simulink library "xrbsComm_r4"  (Simulink 7.1)
PreLoadFcn:
  | warning('off','MATLAB:mex:deprecatedExtension');xlmeta;com.xilinx.sysgen.util.StrategyUtil.loadAllStrategyNames();
undefined symbols (not defined in the file or in its folder): calc_path_data, gcbh, mfcm_matrix_rom, oct2dec, xlBlockLoadCallback
libraries: xbsIndex_r4 x851, mfcm_block_lib_v1 x5, xrbsComm_r4 x1, mfcm_misc_lib_v1 x1
(part 6 of 8)

== system xrbsComm_r4/White Gaussian  Noise Generator/Box-Muller1/f/lfsr_17_2/x1/ASR ==
  din : Inport  OutDataType=sfix(16)  OutScaling=2^0
  Addressable Shift Register : xbsIndex_r4/Addressable Shift Register  infer_latency=off  depth=asr_length  initVector=init  en=off  dbl_ovrd=off  use_behavioral_HDL=off  use_rpm=off  block_type=addrsr
      settings: infoedit="Delay of configurable length.  Any element in the delay line can be addressed and driven onto the output port.<P><P>Hardware notes: Implemented using SRL16s.  If a Virtex-II device is used, multiple SRLC16s are cascaded together."  xl_area=[0, 0, 0, 0, 0, 0, 0]  block_version=VER_STRING_GOES_HERE
  Constant1 : xbsIndex_r4/Constant  arith_type=Unsigned  const=asr_length-1  n_bits=size(dec2bin(asr_length-1),2)  bin_pt=0  explicit_period=off  period=1  equ=P=C  opselect=C  inp2=PCIN>>17  opr=+  inp1=P  carry=CIN  dbl_ovrd=off  block_type=constant
      settings: block_version=VER_STRING_GOES_HERE
  dout : Outport  OutDataType=sfix(16)  OutScaling=2^0
  wires:
  Constant1/1 -> Addressable Shift Register/2
  Addressable Shift Register/1 -> dout/1
  din/1 -> Addressable Shift Register/1

== system xrbsComm_r4/White Gaussian  Noise Generator/Box-Muller1/f/lfsr_17_2/x5/ASR ==
  din : Inport  OutDataType=sfix(16)  OutScaling=2^0
  Addressable Shift Register : xbsIndex_r4/Addressable Shift Register  infer_latency=off  depth=asr_length  initVector=init  en=off  dbl_ovrd=off  use_behavioral_HDL=off  use_rpm=off  block_type=addrsr
      settings: infoedit="Delay of configurable length.  Any element in the delay line can be addressed and driven onto the output port.<P><P>Hardware notes: Implemented using SRL16s.  If a Virtex-II device is used, multiple SRLC16s are cascaded together."  xl_area=[0, 0, 0, 0, 0, 0, 0]  block_version=VER_STRING_GOES_HERE
  Constant : xbsIndex_r4/Constant  arith_type=Unsigned  const=asr_length-1  n_bits=size(dec2bin(asr_length-1),2)  bin_pt=0  explicit_period=off  period=1  equ=P=C  opselect=C  inp2=PCIN>>17  opr=+  inp1=P  carry=CIN  dbl_ovrd=off  block_type=constant
      settings: block_version=VER_STRING_GOES_HERE
  dout : Outport  OutDataType=sfix(16)  OutScaling=2^0
  wires:
  Constant/1 -> Addressable Shift Register/2
  Addressable Shift Register/1 -> dout/1
  din/1 -> Addressable Shift Register/1

== system xrbsComm_r4/White Gaussian  Noise Generator/Box-Muller1/f/lfsr_17_2/x6/ASR ==
  din : Inport  OutDataType=sfix(16)  OutScaling=2^0
  Addressable Shift Register : xbsIndex_r4/Addressable Shift Register  infer_latency=off  depth=asr_length  initVector=init  en=off  dbl_ovrd=off  use_behavioral_HDL=off  use_rpm=off  block_type=addrsr
      settings: infoedit="Delay of configurable length.  Any element in the delay line can be addressed and driven onto the output port.<P><P>Hardware notes: Implemented using SRL16s.  If a Virtex-II device is used, multiple SRLC16s are cascaded together."  xl_area=[0, 0, 0, 0, 0, 0, 0]  block_version=VER_STRING_GOES_HERE
  Constant : xbsIndex_r4/Constant  arith_type=Unsigned  const=asr_length-1  n_bits=size(dec2bin(asr_length-1),2)  bin_pt=0  explicit_period=off  period=1  equ=P=C  opselect=C  inp2=PCIN>>17  opr=+  inp1=P  carry=CIN  dbl_ovrd=off  block_type=constant
      settings: block_version=VER_STRING_GOES_HERE
  dout : Outport  OutDataType=sfix(16)  OutScaling=2^0
  wires:
  Constant/1 -> Addressable Shift Register/2
  Addressable Shift Register/1 -> dout/1
  din/1 -> Addressable Shift Register/1

== system xrbsComm_r4/White Gaussian  Noise Generator/Box-Muller1/f/lfsr_17_2/x7/ASR ==
  din : Inport  OutDataType=sfix(16)  OutScaling=2^0
  Addressable Shift Register : xbsIndex_r4/Addressable Shift Register  infer_latency=off  depth=asr_length  initVector=init  en=off  dbl_ovrd=off  use_behavioral_HDL=off  use_rpm=off  block_type=addrsr
      settings: infoedit="Delay of configurable length.  Any element in the delay line can be addressed and driven onto the output port.<P><P>Hardware notes: Implemented using SRL16s.  If a Virtex-II device is used, multiple SRLC16s are cascaded together."  xl_area=[0, 0, 0, 0, 0, 0, 0]  block_version=VER_STRING_GOES_HERE
  Constant : xbsIndex_r4/Constant  arith_type=Unsigned  const=asr_length-1  n_bits=size(dec2bin(asr_length-1),2)  bin_pt=0  explicit_period=off  period=1  equ=P=C  opselect=C  inp2=PCIN>>17  opr=+  inp1=P  carry=CIN  dbl_ovrd=off  block_type=constant
      settings: block_version=VER_STRING_GOES_HERE
  dout : Outport  OutDataType=sfix(16)  OutScaling=2^0
  wires:
  Constant/1 -> Addressable Shift Register/2
  Addressable Shift Register/1 -> dout/1
  din/1 -> Addressable Shift Register/1

== system xrbsComm_r4/White Gaussian  Noise Generator/Box-Muller1/f/lfsr_25_1/x1/ASR ==
  din : Inport  OutDataType=sfix(16)  OutScaling=2^0
  Addressable Shift Register : xbsIndex_r4/Addressable Shift Register  infer_latency=off  depth=asr_length  initVector=init  en=off  dbl_ovrd=off  use_behavioral_HDL=off  use_rpm=off  block_type=addrsr
      settings: infoedit="Delay of configurable length.  Any element in the delay line can be addressed and driven onto the output port.<P><P>Hardware notes: Implemented using SRL16s.  If a Virtex-II device is used, multiple SRLC16s are cascaded together."  xl_area=[0, 0, 0, 0, 0, 0, 0]  block_version=VER_STRING_GOES_HERE
  Constant1 : xbsIndex_r4/Constant  arith_type=Unsigned  const=asr_length-1  n_bits=size(dec2bin(asr_length-1),2)  bin_pt=0  explicit_period=off  period=1  equ=P=C  opselect=C  inp2=PCIN>>17  opr=+  inp1=P  carry=CIN  dbl_ovrd=off  block_type=constant
      settings: block_version=VER_STRING_GOES_HERE
  dout : Outport  OutDataType=sfix(16)  OutScaling=2^0
  wires:
  Constant1/1 -> Addressable Shift Register/2
  Addressable Shift Register/1 -> dout/1
  din/1 -> Addressable Shift Register/1

== system xrbsComm_r4/White Gaussian  Noise Generator/Box-Muller1/f/lfsr_25_1/x5/ASR ==
  din : Inport  OutDataType=sfix(16)  OutScaling=2^0
  Addressable Shift Register : xbsIndex_r4/Addressable Shift Register  infer_latency=off  depth=asr_length  initVector=init  en=off  dbl_ovrd=off  use_behavioral_HDL=off  use_rpm=off  block_type=addrsr
      settings: infoedit="Delay of configurable length.  Any element in the delay line can be addressed and driven onto the output port.<P><P>Hardware notes: Implemented using SRL16s.  If a Virtex-II device is used, multiple SRLC16s are cascaded together."  xl_area=[0, 0, 0, 0, 0, 0, 0]  block_version=VER_STRING_GOES_HERE
  Constant1 : xbsIndex_r4/Constant  arith_type=Unsigned  const=asr_length-1  n_bits=size(dec2bin(asr_length-1),2)  bin_pt=0  explicit_period=off  period=1  equ=P=C  opselect=C  inp2=PCIN>>17  opr=+  inp1=P  carry=CIN  dbl_ovrd=off  block_type=constant
      settings: block_version=VER_STRING_GOES_HERE
  dout : Outport  OutDataType=sfix(16)  OutScaling=2^0
  wires:
  Constant1/1 -> Addressable Shift Register/2
  Addressable Shift Register/1 -> dout/1
  din/1 -> Addressable Shift Register/1

== system xrbsComm_r4/White Gaussian  Noise Generator/Box-Muller1/f/lfsr_25_1/x6/ASR ==
  din : Inport  OutDataType=sfix(16)  OutScaling=2^0
  Addressable Shift Register : xbsIndex_r4/Addressable Shift Register  infer_latency=off  depth=asr_length  initVector=init  en=off  dbl_ovrd=off  use_behavioral_HDL=off  use_rpm=off  block_type=addrsr
      settings: infoedit="Delay of configurable length.  Any element in the delay line can be addressed and driven onto the output port.<P><P>Hardware notes: Implemented using SRL16s.  If a Virtex-II device is used, multiple SRLC16s are cascaded together."  xl_area=[0, 0, 0, 0, 0, 0, 0]  block_version=VER_STRING_GOES_HERE
  Constant1 : xbsIndex_r4/Constant  arith_type=Unsigned  const=asr_length-1  n_bits=size(dec2bin(asr_length-1),2)  bin_pt=0  explicit_period=off  period=1  equ=P=C  opselect=C  inp2=PCIN>>17  opr=+  inp1=P  carry=CIN  dbl_ovrd=off  block_type=constant
      settings: block_version=VER_STRING_GOES_HERE
  dout : Outport  OutDataType=sfix(16)  OutScaling=2^0
  wires:
  Constant1/1 -> Addressable Shift Register/2
  Addressable Shift Register/1 -> dout/1
  din/1 -> Addressable Shift Register/1

== system xrbsComm_r4/White Gaussian  Noise Generator/Box-Muller1/f/lfsr_25_1/x7/ASR ==
  din : Inport  OutDataType=sfix(16)  OutScaling=2^0
  Addressable Shift Register : xbsIndex_r4/Addressable Shift Register  infer_latency=off  depth=asr_length  initVector=init  en=off  dbl_ovrd=off  use_behavioral_HDL=off  use_rpm=off  block_type=addrsr
      settings: infoedit="Delay of configurable length.  Any element in the delay line can be addressed and driven onto the output port.<P><P>Hardware notes: Implemented using SRL16s.  If a Virtex-II device is used, multiple SRLC16s are cascaded together."  xl_area=[0, 0, 0, 0, 0, 0, 0]  block_version=VER_STRING_GOES_HERE
  Constant1 : xbsIndex_r4/Constant  arith_type=Unsigned  const=asr_length-1  n_bits=size(dec2bin(asr_length-1),2)  bin_pt=0  explicit_period=off  period=1  equ=P=C  opselect=C  inp2=PCIN>>17  opr=+  inp1=P  carry=CIN  dbl_ovrd=off  block_type=constant
      settings: block_version=VER_STRING_GOES_HERE
  dout : Outport  OutDataType=sfix(16)  OutScaling=2^0
  wires:
  Constant1/1 -> Addressable Shift Register/2
  Addressable Shift Register/1 -> dout/1
  din/1 -> Addressable Shift Register/1

== system xrbsComm_r4/White Gaussian  Noise Generator/Box-Muller1/f/lfsr_29_2/x5/ASR ==
  din : Inport  OutDataType=sfix(16)  OutScaling=2^0
  Addressable Shift Register : xbsIndex_r4/Addressable Shift Register  infer_latency=off  depth=asr_length  initVector=init  en=off  dbl_ovrd=off  use_behavioral_HDL=off  use_rpm=off  block_type=addrsr
      settings: infoedit="Delay of configurable length.  Any element in the delay line can be addressed and driven onto the output port.<P><P>Hardware notes: Implemented using SRL16s.  If a Virtex-II device is used, multiple SRLC16s are cascaded together."  xl_area=[0, 0, 0, 0, 0, 0, 0]  block_version=VER_STRING_GOES_HERE
  Constant1 : xbsIndex_r4/Constant  arith_type=Unsigned  const=asr_length-1  n_bits=size(dec2bin(asr_length-1),2)  bin_pt=0  explicit_period=off  period=1  equ=P=C  opselect=C  inp2=PCIN>>17  opr=+  inp1=P  carry=CIN  dbl_ovrd=off  block_type=constant
      settings: block_version=VER_STRING_GOES_HERE
  dout : Outport  OutDataType=sfix(16)  OutScaling=2^0
  wires:
  Constant1/1 -> Addressable Shift Register/2
  Addressable Shift Register/1 -> dout/1
  din/1 -> Addressable Shift Register/1

== system xrbsComm_r4/White Gaussian  Noise Generator/Box-Muller1/f/lfsr_29_2/x6/ASR ==
  din : Inport  OutDataType=sfix(16)  OutScaling=2^0
  Addressable Shift Register : xbsIndex_r4/Addressable Shift Register  infer_latency=off  depth=asr_length  initVector=init  en=off  dbl_ovrd=off  use_behavioral_HDL=off  use_rpm=off  block_type=addrsr
      settings: infoedit="Delay of configurable length.  Any element in the delay line can be addressed and driven onto the output port.<P><P>Hardware notes: Implemented using SRL16s.  If a Virtex-II device is used, multiple SRLC16s are cascaded together."  xl_area=[0, 0, 0, 0, 0, 0, 0]  block_version=VER_STRING_GOES_HERE
  Constant1 : xbsIndex_r4/Constant  arith_type=Unsigned  const=asr_length-1  n_bits=size(dec2bin(asr_length-1),2)  bin_pt=0  explicit_period=off  period=1  equ=P=C  opselect=C  inp2=PCIN>>17  opr=+  inp1=P  carry=CIN  dbl_ovrd=off  block_type=constant
      settings: block_version=VER_STRING_GOES_HERE
  dout : Outport  OutDataType=sfix(16)  OutScaling=2^0
  wires:
  Constant1/1 -> Addressable Shift Register/2
  Addressable Shift Register/1 -> dout/1
  din/1 -> Addressable Shift Register/1

== system xrbsComm_r4/White Gaussian  Noise Generator/Box-Muller1/f/lfsr_29_2/x7/ASR ==
  din : Inport  OutDataType=sfix(16)  OutScaling=2^0
  Addressable Shift Register : xbsIndex_r4/Addressable Shift Register  infer_latency=off  depth=asr_length  initVector=init  en=off  dbl_ovrd=off  use_behavioral_HDL=off  use_rpm=off  block_type=addrsr
      settings: infoedit="Delay of configurable length.  Any element in the delay line can be addressed and driven onto the output port.<P><P>Hardware notes: Implemented using SRL16s.  If a Virtex-II device is used, multiple SRLC16s are cascaded together."  xl_area=[0, 0, 0, 0, 0, 0, 0]  block_version=VER_STRING_GOES_HERE
  Constant1 : xbsIndex_r4/Constant  arith_type=Unsigned  const=asr_length-1  n_bits=size(dec2bin(asr_length-1),2)  bin_pt=0  explicit_period=off  period=1  equ=P=C  opselect=C  inp2=PCIN>>17  opr=+  inp1=P  carry=CIN  dbl_ovrd=off  block_type=constant
      settings: block_version=VER_STRING_GOES_HERE
  dout : Outport  OutDataType=sfix(16)  OutScaling=2^0
  wires:
  Constant1/1 -> Addressable Shift Register/2
  Addressable Shift Register/1 -> dout/1
  din/1 -> Addressable Shift Register/1

== system xrbsComm_r4/White Gaussian  Noise Generator/Box-Muller1/f/lfsr_29_2/x8/ASR ==
  din : Inport  OutDataType=sfix(16)  OutScaling=2^0
  Addressable Shift Register : xbsIndex_r4/Addressable Shift Register  infer_latency=off  depth=asr_length  initVector=init  en=off  dbl_ovrd=off  use_behavioral_HDL=off  use_rpm=off  block_type=addrsr
      settings: infoedit="Delay of configurable length.  Any element in the delay line can be addressed and driven onto the output port.<P><P>Hardware notes: Implemented using SRL16s.  If a Virtex-II device is used, multiple SRLC16s are cascaded together."  xl_area=[0, 0, 0, 0, 0, 0, 0]  block_version=VER_STRING_GOES_HERE
  Constant1 : xbsIndex_r4/Constant  arith_type=Unsigned  const=asr_length-1  n_bits=size(dec2bin(asr_length-1),2)  bin_pt=0  explicit_period=off  period=1  equ=P=C  opselect=C  inp2=PCIN>>17  opr=+  inp1=P  carry=CIN  dbl_ovrd=off  block_type=constant
      settings: block_version=VER_STRING_GOES_HERE
  dout : Outport  OutDataType=sfix(16)  OutScaling=2^0
  wires:
  Constant1/1 -> Addressable Shift Register/2
  Addressable Shift Register/1 -> dout/1
  din/1 -> Addressable Shift Register/1

== system xrbsComm_r4/White Gaussian  Noise Generator/Box-Muller1/f/lfsr_31_2/x5/ASR ==
  din : Inport  OutDataType=sfix(16)  OutScaling=2^0
  Addressable Shift Register : xbsIndex_r4/Addressable Shift Register  infer_latency=off  depth=asr_length  initVector=init  en=off  dbl_ovrd=off  use_behavioral_HDL=off  use_rpm=off  block_type=addrsr
      settings: infoedit="Delay of configurable length.  Any element in the delay line can be addressed and driven onto the output port.<P><P>Hardware notes: Implemented using SRL16s.  If a Virtex-II device is used, multiple SRLC16s are cascaded together."  xl_area=[0, 0, 0, 0, 0, 0, 0]  block_version=VER_STRING_GOES_HERE
  Constant1 : xbsIndex_r4/Constant  arith_type=Unsigned  const=asr_length-1  n_bits=size(dec2bin(asr_length-1),2)  bin_pt=0  explicit_period=off  period=1  equ=P=C  opselect=C  inp2=PCIN>>17  opr=+  inp1=P  carry=CIN  dbl_ovrd=off  block_type=constant
      settings: block_version=VER_STRING_GOES_HERE
  dout : Outport  OutDataType=sfix(16)  OutScaling=2^0
  wires:
  Constant1/1 -> Addressable Shift Register/2
  Addressable Shift Register/1 -> dout/1
  din/1 -> Addressable Shift Register/1

== system xrbsComm_r4/White Gaussian  Noise Generator/Box-Muller1/f/lfsr_31_2/x6/ASR ==
  din : Inport  OutDataType=sfix(16)  OutScaling=2^0
  Addressable Shift Register : xbsIndex_r4/Addressable Shift Register  infer_latency=off  depth=asr_length  initVector=init  en=off  dbl_ovrd=off  use_behavioral_HDL=off  use_rpm=off  block_type=addrsr
      settings: infoedit="Delay of configurable length.  Any element in the delay line can be addressed and driven onto the output port.<P><P>Hardware notes: Implemented using SRL16s.  If a Virtex-II device is used, multiple SRLC16s are cascaded together."  xl_area=[0, 0, 0, 0, 0, 0, 0]  block_version=VER_STRING_GOES_HERE
  Constant1 : xbsIndex_r4/Constant  arith_type=Unsigned  const=asr_length-1  n_bits=size(dec2bin(asr_length-1),2)  bin_pt=0  explicit_period=off  period=1  equ=P=C  opselect=C  inp2=PCIN>>17  opr=+  inp1=P  carry=CIN  dbl_ovrd=off  block_type=constant
      settings: block_version=VER_STRING_GOES_HERE
  dout : Outport  OutDataType=sfix(16)  OutScaling=2^0
  wires:
  Constant1/1 -> Addressable Shift Register/2
  Addressable Shift Register/1 -> dout/1
  din/1 -> Addressable Shift Register/1

== system xrbsComm_r4/White Gaussian  Noise Generator/Box-Muller1/f/lfsr_31_2/x7/ASR ==
  din : Inport  OutDataType=sfix(16)  OutScaling=2^0
  Addressable Shift Register : xbsIndex_r4/Addressable Shift Register  infer_latency=off  depth=asr_length  initVector=init  en=off  dbl_ovrd=off  use_behavioral_HDL=off  use_rpm=off  block_type=addrsr
      settings: infoedit="Delay of configurable length.  Any element in the delay line can be addressed and driven onto the output port.<P><P>Hardware notes: Implemented using SRL16s.  If a Virtex-II device is used, multiple SRLC16s are cascaded together."  xl_area=[0, 0, 0, 0, 0, 0, 0]  block_version=VER_STRING_GOES_HERE
  Constant1 : xbsIndex_r4/Constant  arith_type=Unsigned  const=asr_length-1  n_bits=size(dec2bin(asr_length-1),2)  bin_pt=0  explicit_period=off  period=1  equ=P=C  opselect=C  inp2=PCIN>>17  opr=+  inp1=P  carry=CIN  dbl_ovrd=off  block_type=constant
      settings: block_version=VER_STRING_GOES_HERE
  dout : Outport  OutDataType=sfix(16)  OutScaling=2^0
  wires:
  Constant1/1 -> Addressable Shift Register/2
  Addressable Shift Register/1 -> dout/1
  din/1 -> Addressable Shift Register/1

== system xrbsComm_r4/White Gaussian  Noise Generator/Box-Muller1/f/lfsr_31_2/x8/ASR ==
  din : Inport  OutDataType=sfix(16)  OutScaling=2^0
  Addressable Shift Register : xbsIndex_r4/Addressable Shift Register  infer_latency=off  depth=asr_length  initVector=init  en=off  dbl_ovrd=off  use_behavioral_HDL=off  use_rpm=off  block_type=addrsr
      settings: infoedit="Delay of configurable length.  Any element in the delay line can be addressed and driven onto the output port.<P><P>Hardware notes: Implemented using SRL16s.  If a Virtex-II device is used, multiple SRLC16s are cascaded together."  xl_area=[0, 0, 0, 0, 0, 0, 0]  block_version=VER_STRING_GOES_HERE
  Constant1 : xbsIndex_r4/Constant  arith_type=Unsigned  const=asr_length-1  n_bits=size(dec2bin(asr_length-1),2)  bin_pt=0  explicit_period=off  period=1  equ=P=C  opselect=C  inp2=PCIN>>17  opr=+  inp1=P  carry=CIN  dbl_ovrd=off  block_type=constant
      settings: block_version=VER_STRING_GOES_HERE
  dout : Outport  OutDataType=sfix(16)  OutScaling=2^0
  wires:
  Constant1/1 -> Addressable Shift Register/2
  Addressable Shift Register/1 -> dout/1
  din/1 -> Addressable Shift Register/1

== system xrbsComm_r4/White Gaussian  Noise Generator/Box-Muller1/f/lfsr_41_2/x1/ASR ==
  din : Inport  OutDataType=sfix(16)  OutScaling=2^0
  Addressable Shift Register : xbsIndex_r4/Addressable Shift Register  infer_latency=off  depth=asr_length  initVector=init  en=off  dbl_ovrd=off  use_behavioral_HDL=off  use_rpm=off  block_type=addrsr
      settings: infoedit="Delay of configurable length.  Any element in the delay line can be addressed and driven onto the output port.<P><P>Hardware notes: Implemented using SRL16s.  If a Virtex-II device is used, multiple SRLC16s are cascaded together."  xl_area=[0, 0, 0, 0, 0, 0, 0]  block_version=VER_STRING_GOES_HERE
  Constant1 : xbsIndex_r4/Constant  arith_type=Unsigned  const=asr_length-1  n_bits=size(dec2bin(asr_length-1),2)  bin_pt=0  explicit_period=off  period=1  equ=P=C  opselect=C  inp2=PCIN>>17  opr=+  inp1=P  carry=CIN  dbl_ovrd=off  block_type=constant
      settings: block_version=VER_STRING_GOES_HERE
  dout : Outport  OutDataType=sfix(16)  OutScaling=2^0
  wires:
  Constant1/1 -> Addressable Shift Register/2
  Addressable Shift Register/1 -> dout/1
  din/1 -> Addressable Shift Register/1

== system xrbsComm_r4/White Gaussian  Noise Generator/Box-Muller1/f/lfsr_41_2/x5/ASR ==
  din : Inport  OutDataType=sfix(16)  OutScaling=2^0
  Addressable Shift Register : xbsIndex_r4/Addressable Shift Register  infer_latency=off  depth=asr_length  initVector=init  en=off  dbl_ovrd=off  use_behavioral_HDL=off  use_rpm=off  block_type=addrsr
      settings: infoedit="Delay of configurable length.  Any element in the delay line can be addressed and driven onto the output port.<P><P>Hardware notes: Implemented using SRL16s.  If a Virtex-II device is used, multiple SRLC16s are cascaded together."  xl_area=[0, 0, 0, 0, 0, 0, 0]  block_version=VER_STRING_GOES_HERE
  Constant1 : xbsIndex_r4/Constant  arith_type=Unsigned  const=asr_length-1  n_bits=size(dec2bin(asr_length-1),2)  bin_pt=0  explicit_period=off  period=1  equ=P=C  opselect=C  inp2=PCIN>>17  opr=+  inp1=P  carry=CIN  dbl_ovrd=off  block_type=constant
      settings: block_version=VER_STRING_GOES_HERE
  dout : Outport  OutDataType=sfix(16)  OutScaling=2^0
  wires:
  Constant1/1 -> Addressable Shift Register/2
  Addressable Shift Register/1 -> dout/1
  din/1 -> Addressable Shift Register/1

== system xrbsComm_r4/White Gaussian  Noise Generator/Box-Muller1/f/lfsr_41_2/x6/ASR ==
  din : Inport  OutDataType=sfix(16)  OutScaling=2^0
  Addressable Shift Register : xbsIndex_r4/Addressable Shift Register  infer_latency=off  depth=asr_length  initVector=init  en=off  dbl_ovrd=off  use_behavioral_HDL=off  use_rpm=off  block_type=addrsr
      settings: infoedit="Delay of configurable length.  Any element in the delay line can be addressed and driven onto the output port.<P><P>Hardware notes: Implemented using SRL16s.  If a Virtex-II device is used, multiple SRLC16s are cascaded together."  xl_area=[0, 0, 0, 0, 0, 0, 0]  block_version=VER_STRING_GOES_HERE
  Constant1 : xbsIndex_r4/Constant  arith_type=Unsigned  const=asr_length-1  n_bits=size(dec2bin(asr_length-1),2)  bin_pt=0  explicit_period=off  period=1  equ=P=C  opselect=C  inp2=PCIN>>17  opr=+  inp1=P  carry=CIN  dbl_ovrd=off  block_type=constant
      settings: block_version=VER_STRING_GOES_HERE
  dout : Outport  OutDataType=sfix(16)  OutScaling=2^0
  wires:
  Constant1/1 -> Addressable Shift Register/2
  Addressable Shift Register/1 -> dout/1
  din/1 -> Addressable Shift Register/1

== system xrbsComm_r4/White Gaussian  Noise Generator/Box-Muller1/f/lfsr_41_2/x7/ASR ==
  din : Inport  OutDataType=sfix(16)  OutScaling=2^0
  Addressable Shift Register : xbsIndex_r4/Addressable Shift Register  infer_latency=off  depth=asr_length  initVector=init  en=off  dbl_ovrd=off  use_behavioral_HDL=off  use_rpm=off  block_type=addrsr
      settings: infoedit="Delay of configurable length.  Any element in the delay line can be addressed and driven onto the output port.<P><P>Hardware notes: Implemented using SRL16s.  If a Virtex-II device is used, multiple SRLC16s are cascaded together."  xl_area=[0, 0, 0, 0, 0, 0, 0]  block_version=VER_STRING_GOES_HERE
  Constant1 : xbsIndex_r4/Constant  arith_type=Unsigned  const=asr_length-1  n_bits=size(dec2bin(asr_length-1),2)  bin_pt=0  explicit_period=off  period=1  equ=P=C  opselect=C  inp2=PCIN>>17  opr=+  inp1=P  carry=CIN  dbl_ovrd=off  block_type=constant
      settings: block_version=VER_STRING_GOES_HERE
  dout : Outport  OutDataType=sfix(16)  OutScaling=2^0
  wires:
  Constant1/1 -> Addressable Shift Register/2
  Addressable Shift Register/1 -> dout/1
  din/1 -> Addressable Shift Register/1

== system xrbsComm_r4/White Gaussian  Noise Generator/Box-Muller1/g/lfsr_47_5/x10/ASR ==
  din : Inport  OutDataType=sfix(16)  OutScaling=2^0
  Addressable Shift Register : xbsIndex_r4/Addressable Shift Register  infer_latency=off  depth=asr_length  initVector=init  en=off  dbl_ovrd=off  use_behavioral_HDL=off  use_rpm=off  block_type=addrsr
      settings: infoedit="Delay of configurable length.  Any element in the delay line can be addressed and driven onto the output port.<P><P>Hardware notes: Implemented using SRL16s.  If a Virtex-II device is used, multiple SRLC16s are cascaded together."  xl_area=[0, 0, 0, 0, 0, 0, 0]  block_version=VER_STRING_GOES_HERE
  Constant1 : xbsIndex_r4/Constant  arith_type=Unsigned  const=asr_length-1  n_bits=size(dec2bin(asr_length-1),2)  bin_pt=0  explicit_period=off  period=1  equ=P=C  opselect=C  inp2=PCIN>>17  opr=+  inp1=P  carry=CIN  dbl_ovrd=off  block_type=constant
      settings: block_version=VER_STRING_GOES_HERE
  dout : Outport  OutDataType=sfix(16)  OutScaling=2^0
  wires:
  Constant1/1 -> Addressable Shift Register/2
  Addressable Shift Register/1 -> dout/1
  din/1 -> Addressable Shift Register/1

== system xrbsComm_r4/White Gaussian  Noise Generator/Box-Muller1/g/lfsr_47_5/x11/ASR ==
  din : Inport  OutDataType=sfix(16)  OutScaling=2^0
  Addressable Shift Register : xbsIndex_r4/Addressable Shift Register  infer_latency=off  depth=asr_length  initVector=init  en=off  dbl_ovrd=off  use_behavioral_HDL=off  use_rpm=off  block_type=addrsr
      settings: infoedit="Delay of configurable length.  Any element in the delay line can be addressed and driven onto the output port.<P><P>Hardware notes: Implemented using SRL16s.  If a Virtex-II device is used, multiple SRLC16s are cascaded together."  xl_area=[0, 0, 0, 0, 0, 0, 0]  block_version=VER_STRING_GOES_HERE
  Constant1 : xbsIndex_r4/Constant  arith_type=Unsigned  const=asr_length-1  n_bits=size(dec2bin(asr_length-1),2)  bin_pt=0  explicit_period=off  period=1  equ=P=C  opselect=C  inp2=PCIN>>17  opr=+  inp1=P  carry=CIN  dbl_ovrd=off  block_type=constant
      settings: block_version=VER_STRING_GOES_HERE
  dout : Outport  OutDataType=sfix(16)  OutScaling=2^0
  wires:
  Constant1/1 -> Addressable Shift Register/2
  Addressable Shift Register/1 -> dout/1
  din/1 -> Addressable Shift Register/1

== system xrbsComm_r4/White Gaussian  Noise Generator/Box-Muller1/g/lfsr_47_5/x12/ASR ==
  din : Inport  OutDataType=sfix(16)  OutScaling=2^0
  Addressable Shift Register : xbsIndex_r4/Addressable Shift Register  infer_latency=off  depth=asr_length  initVector=init  en=off  dbl_ovrd=off  use_behavioral_HDL=off  use_rpm=off  block_type=addrsr
      settings: infoedit="Delay of configurable length.  Any element in the delay line can be addressed and driven onto the output port.<P><P>Hardware notes: Implemented using SRL16s.  If a Virtex-II device is used, multiple SRLC16s are cascaded together."  xl_area=[0, 0, 0, 0, 0, 0, 0]  block_version=VER_STRING_GOES_HERE
  Constant1 : xbsIndex_r4/Constant  arith_type=Unsigned  const=asr_length-1  n_bits=size(dec2bin(asr_length-1),2)  bin_pt=0  explicit_period=off  period=1  equ=P=C  opselect=C  inp2=PCIN>>17  opr=+  inp1=P  carry=CIN  dbl_ovrd=off  block_type=constant
      settings: block_version=VER_STRING_GOES_HERE
  dout : Outport  OutDataType=sfix(16)  OutScaling=2^0
  wires:
  Constant1/1 -> Addressable Shift Register/2
  Addressable Shift Register/1 -> dout/1
  din/1 -> Addressable Shift Register/1

== system xrbsComm_r4/White Gaussian  Noise Generator/Box-Muller1/g/lfsr_47_5/x13/ASR ==
  din : Inport  OutDataType=sfix(16)  OutScaling=2^0
  Addressable Shift Register : xbsIndex_r4/Addressable Shift Register  infer_latency=off  depth=asr_length  initVector=init  en=off  dbl_ovrd=off  use_behavioral_HDL=off  use_rpm=off  block_type=addrsr
      settings: infoedit="Delay of configurable length.  Any element in the delay line can be addressed and driven onto the output port.<P><P>Hardware notes: Implemented using SRL16s.  If a Virtex-II device is used, multiple SRLC16s are cascaded together."  xl_area=[0, 0, 0, 0, 0, 0, 0]  block_version=VER_STRING_GOES_HERE
  Constant1 : xbsIndex_r4/Constant  arith_type=Unsigned  const=asr_length-1  n_bits=size(dec2bin(asr_length-1),2)  bin_pt=0  explicit_period=off  period=1  equ=P=C  opselect=C  inp2=PCIN>>17  opr=+  inp1=P  carry=CIN  dbl_ovrd=off  block_type=constant
      settings: block_version=VER_STRING_GOES_HERE
  dout : Outport  OutDataType=sfix(16)  OutScaling=2^0
  wires:
  Constant1/1 -> Addressable Shift Register/2
  Addressable Shift Register/1 -> dout/1
  din/1 -> Addressable Shift Register/1

== system xrbsComm_r4/White Gaussian  Noise Generator/Box-Muller1/g/lfsr_47_5/x14/ASR ==
  din : Inport  OutDataType=sfix(16)  OutScaling=2^0
  Addressable Shift Register : xbsIndex_r4/Addressable Shift Register  infer_latency=off  depth=asr_length  initVector=init  en=off  dbl_ovrd=off  use_behavioral_HDL=off  use_rpm=off  block_type=addrsr
      settings: infoedit="Delay of configurable length.  Any element in the delay line can be addressed and driven onto the output port.<P><P>Hardware notes: Implemented using SRL16s.  If a Virtex-II device is used, multiple SRLC16s are cascaded together."  xl_area=[0, 0, 0, 0, 0, 0, 0]  block_version=VER_STRING_GOES_HERE
  Constant1 : xbsIndex_r4/Constant  arith_type=Unsigned  const=asr_length-1  n_bits=size(dec2bin(asr_length-1),2)  bin_pt=0  explicit_period=off  period=1  equ=P=C  opselect=C  inp2=PCIN>>17  opr=+  inp1=P  carry=CIN  dbl_ovrd=off  block_type=constant
      settings: block_version=VER_STRING_GOES_HERE
  dout : Outport  OutDataType=sfix(16)  OutScaling=2^0
  wires:
  Constant1/1 -> Addressable Shift Register/2
  Addressable Shift Register/1 -> dout/1
  din/1 -> Addressable Shift Register/1

== system xrbsComm_r4/White Gaussian  Noise Generator/Box-Muller1/g/lfsr_47_5/x15/ASR ==
  din : Inport  OutDataType=sfix(16)  OutScaling=2^0
  Addressable Shift Register : xbsIndex_r4/Addressable Shift Register  infer_latency=off  depth=asr_length  initVector=init  en=off  dbl_ovrd=off  use_behavioral_HDL=off  use_rpm=off  block_type=addrsr
      settings: infoedit="Delay of configurable length.  Any element in the delay line can be addressed and driven onto the output port.<P><P>Hardware notes: Implemented using SRL16s.  If a Virtex-II device is used, multiple SRLC16s are cascaded together."  xl_area=[0, 0, 0, 0, 0, 0, 0]  block_version=VER_STRING_GOES_HERE
  Constant1 : xbsIndex_r4/Constant  arith_type=Unsigned  const=asr_length-1  n_bits=size(dec2bin(asr_length-1),2)  bin_pt=0  explicit_period=off  period=1  equ=P=C  opselect=C  inp2=PCIN>>17  opr=+  inp1=P  carry=CIN  dbl_ovrd=off  block_type=constant
      settings: block_version=VER_STRING_GOES_HERE
  dout : Outport  OutDataType=sfix(16)  OutScaling=2^0
  wires:
  Constant1/1 -> Addressable Shift Register/2
  Addressable Shift Register/1 -> dout/1
  din/1 -> Addressable Shift Register/1

== system xrbsComm_r4/White Gaussian  Noise Generator/Box-Muller1/g/lfsr_47_5/x16/ASR ==
  din : Inport  OutDataType=sfix(16)  OutScaling=2^0
  Addressable Shift Register : xbsIndex_r4/Addressable Shift Register  infer_latency=off  depth=asr_length  initVector=init  en=off  dbl_ovrd=off  use_behavioral_HDL=off  use_rpm=off  block_type=addrsr
      settings: infoedit="Delay of configurable length.  Any element in the delay line can be addressed and driven onto the output port.<P><P>Hardware notes: Implemented using SRL16s.  If a Virtex-II device is used, multiple SRLC16s are cascaded together."  xl_area=[0, 0, 0, 0, 0, 0, 0]  block_version=VER_STRING_GOES_HERE
  Constant1 : xbsIndex_r4/Constant  arith_type=Unsigned  const=asr_length-1  n_bits=size(dec2bin(asr_length-1),2)  bin_pt=0  explicit_period=off  period=1  equ=P=C  opselect=C  inp2=PCIN>>17  opr=+  inp1=P  carry=CIN  dbl_ovrd=off  block_type=constant
      settings: block_version=VER_STRING_GOES_HERE
  dout : Outport  OutDataType=sfix(16)  OutScaling=2^0
  wires:
  Constant1/1 -> Addressable Shift Register/2
  Addressable Shift Register/1 -> dout/1
  din/1 -> Addressable Shift Register/1

== system xrbsComm_r4/White Gaussian  Noise Generator/Box-Muller1/g/lfsr_47_5/x9/ASR ==
  din : Inport  OutDataType=sfix(16)  OutScaling=2^0
  Addressable Shift Register : xbsIndex_r4/Addressable Shift Register  infer_latency=off  depth=asr_length  initVector=init  en=off  dbl_ovrd=off  use_behavioral_HDL=off  use_rpm=off  block_type=addrsr
      settings: infoedit="Delay of configurable length.  Any element in the delay line can be addressed and driven onto the output port.<P><P>Hardware notes: Implemented using SRL16s.  If a Virtex-II device is used, multiple SRLC16s are cascaded together."  xl_area=[0, 0, 0, 0, 0, 0, 0]  block_version=VER_STRING_GOES_HERE
  Constant1 : xbsIndex_r4/Constant  arith_type=Unsigned  const=asr_length-1  n_bits=size(dec2bin(asr_length-1),2)  bin_pt=0  explicit_period=off  period=1  equ=P=C  opselect=C  inp2=PCIN>>17  opr=+  inp1=P  carry=CIN  dbl_ovrd=off  block_type=constant
      settings: block_version=VER_STRING_GOES_HERE
  dout : Outport  OutDataType=sfix(16)  OutScaling=2^0
  wires:
  Constant1/1 -> Addressable Shift Register/2
  Addressable Shift Register/1 -> dout/1
  din/1 -> Addressable Shift Register/1

== system xrbsComm_r4/White Gaussian  Noise Generator/Box-Muller2/fr1/lfsr_17_2/x1/ASR ==
  din : Inport  OutDataType=sfix(16)  OutScaling=2^0
  Addressable Shift Register : xbsIndex_r4/Addressable Shift Register  infer_latency=off  depth=asr_length  initVector=init  en=off  dbl_ovrd=off  use_behavioral_HDL=off  use_rpm=off  block_type=addrsr
      settings: infoedit="Delay of configurable length.  Any element in the delay line can be addressed and driven onto the output port.<P><P>Hardware notes: Implemented using SRL16s.  If a Virtex-II device is used, multiple SRLC16s are cascaded together."  xl_area=[0, 0, 0, 0, 0, 0, 0]  block_version=VER_STRING_GOES_HERE
  Constant : xbsIndex_r4/Constant  arith_type=Unsigned  const=asr_length-1  n_bits=size(dec2bin(asr_length-1),2)  bin_pt=0  explicit_period=off  period=1  equ=P=C  opselect=C  inp2=PCIN>>17  opr=+  inp1=P  carry=CIN  dbl_ovrd=off  block_type=constant
      settings: block_version=VER_STRING_GOES_HERE
  dout : Outport  OutDataType=sfix(16)  OutScaling=2^0
  wires:
  Constant/1 -> Addressable Shift Register/2
  Addressable Shift Register/1 -> dout/1
  din/1 -> Addressable Shift Register/1

== system xrbsComm_r4/White Gaussian  Noise Generator/Box-Muller2/fr1/lfsr_17_2/x5/ASR ==
  din : Inport  OutDataType=sfix(16)  OutScaling=2^0
  Addressable Shift Register : xbsIndex_r4/Addressable Shift Register  infer_latency=off  depth=asr_length  initVector=init  en=off  dbl_ovrd=off  use_behavioral_HDL=off  use_rpm=off  block_type=addrsr
      settings: infoedit="Delay of configurable length.  Any element in the delay line can be addressed and driven onto the output port.<P><P>Hardware notes: Implemented using SRL16s.  If a Virtex-II device is used, multiple SRLC16s are cascaded together."  xl_area=[0, 0, 0, 0, 0, 0, 0]  block_version=VER_STRING_GOES_HERE
  Constant1 : xbsIndex_r4/Constant  arith_type=Unsigned  const=asr_length-1  n_bits=size(dec2bin(asr_length-1),2)  bin_pt=0  explicit_period=off  period=1  equ=P=C  opselect=C  inp2=PCIN>>17  opr=+  inp1=P  carry=CIN  dbl_ovrd=off  block_type=constant
      settings: block_version=VER_STRING_GOES_HERE
  dout : Outport  OutDataType=sfix(16)  OutScaling=2^0
  wires:
  Constant1/1 -> Addressable Shift Register/2
  Addressable Shift Register/1 -> dout/1
  din/1 -> Addressable Shift Register/1

== system xrbsComm_r4/White Gaussian  Noise Generator/Box-Muller2/fr1/lfsr_17_2/x6/ASR ==
  din : Inport  OutDataType=sfix(16)  OutScaling=2^0
  Addressable Shift Register : xbsIndex_r4/Addressable Shift Register  infer_latency=off  depth=asr_length  initVector=init  en=off  dbl_ovrd=off  use_behavioral_HDL=off  use_rpm=off  block_type=addrsr
      settings: infoedit="Delay of configurable length.  Any element in the delay line can be addressed and driven onto the output port.<P><P>Hardware notes: Implemented using SRL16s.  If a Virtex-II device is used, multiple SRLC16s are cascaded together."  xl_area=[0, 0, 0, 0, 0, 0, 0]  block_version=VER_STRING_GOES_HERE
  Constant1 : xbsIndex_r4/Constant  arith_type=Unsigned  const=asr_length-1  n_bits=size(dec2bin(asr_length-1),2)  bin_pt=0  explicit_period=off  period=1  equ=P=C  opselect=C  inp2=PCIN>>17  opr=+  inp1=P  carry=CIN  dbl_ovrd=off  block_type=constant
      settings: block_version=VER_STRING_GOES_HERE
  dout : Outport  OutDataType=sfix(16)  OutScaling=2^0
  wires:
  Constant1/1 -> Addressable Shift Register/2
  Addressable Shift Register/1 -> dout/1
  din/1 -> Addressable Shift Register/1

== system xrbsComm_r4/White Gaussian  Noise Generator/Box-Muller2/fr1/lfsr_17_2/x7/ASR ==
  din : Inport  OutDataType=sfix(16)  OutScaling=2^0
  Addressable Shift Register : xbsIndex_r4/Addressable Shift Register  infer_latency=off  depth=asr_length  initVector=init  en=off  dbl_ovrd=off  use_behavioral_HDL=off  use_rpm=off  block_type=addrsr
      settings: infoedit="Delay of configurable length.  Any element in the delay line can be addressed and driven onto the output port.<P><P>Hardware notes: Implemented using SRL16s.  If a Virtex-II device is used, multiple SRLC16s are cascaded together."  xl_area=[0, 0, 0, 0, 0, 0, 0]  block_version=VER_STRING_GOES_HERE
  Constant1 : xbsIndex_r4/Constant  arith_type=Unsigned  const=asr_length-1  n_bits=size(dec2bin(asr_length-1),2)  bin_pt=0  explicit_period=off  period=1  equ=P=C  opselect=C  inp2=PCIN>>17  opr=+  inp1=P  carry=CIN  dbl_ovrd=off  block_type=constant
      settings: block_version=VER_STRING_GOES_HERE
  dout : Outport  OutDataType=sfix(16)  OutScaling=2^0
  wires:
  Constant1/1 -> Addressable Shift Register/2
  Addressable Shift Register/1 -> dout/1
  din/1 -> Addressable Shift Register/1

== system xrbsComm_r4/White Gaussian  Noise Generator/Box-Muller2/fr1/lfsr_25_2/x1/ASR ==
  din : Inport  OutDataType=sfix(16)  OutScaling=2^0
  Addressable Shift Register : xbsIndex_r4/Addressable Shift Register  infer_latency=off  depth=asr_length  initVector=init  en=off  dbl_ovrd=off  use_behavioral_HDL=off  use_rpm=off  block_type=addrsr
      settings: infoedit="Delay of configurable length.  Any element in the delay line can be addressed and driven onto the output port.<P><P>Hardware notes: Implemented using SRL16s.  If a Virtex-II device is used, multiple SRLC16s are cascaded together."  xl_area=[0, 0, 0, 0, 0, 0, 0]  block_version=VER_STRING_GOES_HERE
  Constant1 : xbsIndex_r4/Constant  arith_type=Unsigned  const=asr_length-1  n_bits=size(dec2bin(asr_length-1),2)  bin_pt=0  explicit_period=off  period=1  equ=P=C  opselect=C  inp2=PCIN>>17  opr=+  inp1=P  carry=CIN  dbl_ovrd=off  block_type=constant
      settings: block_version=VER_STRING_GOES_HERE
  dout : Outport  OutDataType=sfix(16)  OutScaling=2^0
  wires:
  Constant1/1 -> Addressable Shift Register/2
  Addressable Shift Register/1 -> dout/1
  din/1 -> Addressable Shift Register/1

== system xrbsComm_r4/White Gaussian  Noise Generator/Box-Muller2/fr1/lfsr_25_2/x5/ASR ==
  din : Inport  OutDataType=sfix(16)  OutScaling=2^0
  Addressable Shift Register : xbsIndex_r4/Addressable Shift Register  infer_latency=off  depth=asr_length  initVector=init  en=off  dbl_ovrd=off  use_behavioral_HDL=off  use_rpm=off  block_type=addrsr
      settings: infoedit="Delay of configurable length.  Any element in the delay line can be addressed and driven onto the output port.<P><P>Hardware notes: Implemented using SRL16s.  If a Virtex-II device is used, multiple SRLC16s are cascaded together."  xl_area=[0, 0, 0, 0, 0, 0, 0]  block_version=VER_STRING_GOES_HERE
  Constant1 : xbsIndex_r4/Constant  arith_type=Unsigned  const=asr_length-1  n_bits=size(dec2bin(asr_length-1),2)  bin_pt=0  explicit_period=off  period=1  equ=P=C  opselect=C  inp2=PCIN>>17  opr=+  inp1=P  carry=CIN  dbl_ovrd=off  block_type=constant
      settings: block_version=VER_STRING_GOES_HERE
  dout : Outport  OutDataType=sfix(16)  OutScaling=2^0
  wires:
  Constant1/1 -> Addressable Shift Register/2
  Addressable Shift Register/1 -> dout/1
  din/1 -> Addressable Shift Register/1

== system xrbsComm_r4/White Gaussian  Noise Generator/Box-Muller2/fr1/lfsr_25_2/x6/ASR ==
  din : Inport  OutDataType=sfix(16)  OutScaling=2^0
  Addressable Shift Register : xbsIndex_r4/Addressable Shift Register  infer_latency=off  depth=asr_length  initVector=init  en=off  dbl_ovrd=off  use_behavioral_HDL=off  use_rpm=off  block_type=addrsr
      settings: infoedit="Delay of configurable length.  Any element in the delay line can be addressed and driven onto the output port.<P><P>Hardware notes: Implemented using SRL16s.  If a Virtex-II device is used, multiple SRLC16s are cascaded together."  xl_area=[0, 0, 0, 0, 0, 0, 0]  block_version=VER_STRING_GOES_HERE
  Constant1 : xbsIndex_r4/Constant  arith_type=Unsigned  const=asr_length-1  n_bits=size(dec2bin(asr_length-1),2)  bin_pt=0  explicit_period=off  period=1  equ=P=C  opselect=C  inp2=PCIN>>17  opr=+  inp1=P  carry=CIN  dbl_ovrd=off  block_type=constant
      settings: block_version=VER_STRING_GOES_HERE
  dout : Outport  OutDataType=sfix(16)  OutScaling=2^0
  wires:
  Constant1/1 -> Addressable Shift Register/2
  Addressable Shift Register/1 -> dout/1
  din/1 -> Addressable Shift Register/1

== system xrbsComm_r4/White Gaussian  Noise Generator/Box-Muller2/fr1/lfsr_25_2/x7/ASR ==
  din : Inport  OutDataType=sfix(16)  OutScaling=2^0
  Addressable Shift Register : xbsIndex_r4/Addressable Shift Register  infer_latency=off  depth=asr_length  initVector=init  en=off  dbl_ovrd=off  use_behavioral_HDL=off  use_rpm=off  block_type=addrsr
      settings: infoedit="Delay of configurable length.  Any element in the delay line can be addressed and driven onto the output port.<P><P>Hardware notes: Implemented using SRL16s.  If a Virtex-II device is used, multiple SRLC16s are cascaded together."  xl_area=[0, 0, 0, 0, 0, 0, 0]  block_version=VER_STRING_GOES_HERE
  Constant1 : xbsIndex_r4/Constant  arith_type=Unsigned  const=asr_length-1  n_bits=size(dec2bin(asr_length-1),2)  bin_pt=0  explicit_period=off  period=1  equ=P=C  opselect=C  inp2=PCIN>>17  opr=+  inp1=P  carry=CIN  dbl_ovrd=off  block_type=constant
      settings: block_version=VER_STRING_GOES_HERE
  dout : Outport  OutDataType=sfix(16)  OutScaling=2^0
  wires:
  Constant1/1 -> Addressable Shift Register/2
  Addressable Shift Register/1 -> dout/1
  din/1 -> Addressable Shift Register/1

== system xrbsComm_r4/White Gaussian  Noise Generator/Box-Muller2/fr1/lfsr_29_2/x5/ASR ==
  din : Inport  OutDataType=sfix(16)  OutScaling=2^0
  Addressable Shift Register : xbsIndex_r4/Addressable Shift Register  infer_latency=off  depth=asr_length  initVector=init  en=off  dbl_ovrd=off  use_behavioral_HDL=off  use_rpm=off  block_type=addrsr
      settings: infoedit="Delay of configurable length.  Any element in the delay line can be addressed and driven onto the output port.<P><P>Hardware notes: Implemented using SRL16s.  If a Virtex-II device is used, multiple SRLC16s are cascaded together."  xl_area=[0, 0, 0, 0, 0, 0, 0]  block_version=VER_STRING_GOES_HERE
  Constant1 : xbsIndex_r4/Constant  arith_type=Unsigned  const=asr_length-1  n_bits=size(dec2bin(asr_length-1),2)  bin_pt=0  explicit_period=off  period=1  equ=P=C  opselect=C  inp2=PCIN>>17  opr=+  inp1=P  carry=CIN  dbl_ovrd=off  block_type=constant
      settings: block_version=VER_STRING_GOES_HERE
  dout : Outport  OutDataType=sfix(16)  OutScaling=2^0
  wires:
  Constant1/1 -> Addressable Shift Register/2
  Addressable Shift Register/1 -> dout/1
  din/1 -> Addressable Shift Register/1

== system xrbsComm_r4/White Gaussian  Noise Generator/Box-Muller2/fr1/lfsr_29_2/x6/ASR ==
  din : Inport  OutDataType=sfix(16)  OutScaling=2^0
  Addressable Shift Register : xbsIndex_r4/Addressable Shift Register  infer_latency=off  depth=asr_length  initVector=init  en=off  dbl_ovrd=off  use_behavioral_HDL=off  use_rpm=off  block_type=addrsr
      settings: infoedit="Delay of configurable length.  Any element in the delay line can be addressed and driven onto the output port.<P><P>Hardware notes: Implemented using SRL16s.  If a Virtex-II device is used, multiple SRLC16s are cascaded together."  xl_area=[0, 0, 0, 0, 0, 0, 0]  block_version=VER_STRING_GOES_HERE
  Constant1 : xbsIndex_r4/Constant  arith_type=Unsigned  const=asr_length-1  n_bits=size(dec2bin(asr_length-1),2)  bin_pt=0  explicit_period=off  period=1  equ=P=C  opselect=C  inp2=PCIN>>17  opr=+  inp1=P  carry=CIN  dbl_ovrd=off  block_type=constant
      settings: block_version=VER_STRING_GOES_HERE
  dout : Outport  OutDataType=sfix(16)  OutScaling=2^0
  wires:
  Constant1/1 -> Addressable Shift Register/2
  Addressable Shift Register/1 -> dout/1
  din/1 -> Addressable Shift Register/1

== system xrbsComm_r4/White Gaussian  Noise Generator/Box-Muller2/fr1/lfsr_29_2/x7/ASR ==
  din : Inport  OutDataType=sfix(16)  OutScaling=2^0
  Addressable Shift Register : xbsIndex_r4/Addressable Shift Register  infer_latency=off  depth=asr_length  initVector=init  en=off  dbl_ovrd=off  use_behavioral_HDL=off  use_rpm=off  block_type=addrsr
      settings: infoedit="Delay of configurable length.  Any element in the delay line can be addressed and driven onto the output port.<P><P>Hardware notes: Implemented using SRL16s.  If a Virtex-II device is used, multiple SRLC16s are cascaded together."  xl_area=[0, 0, 0, 0, 0, 0, 0]  block_version=VER_STRING_GOES_HERE
  Constant1 : xbsIndex_r4/Constant  arith_type=Unsigned  const=asr_length-1  n_bits=size(dec2bin(asr_length-1),2)  bin_pt=0  explicit_period=off  period=1  equ=P=C  opselect=C  inp2=PCIN>>17  opr=+  inp1=P  carry=CIN  dbl_ovrd=off  block_type=constant
      settings: block_version=VER_STRING_GOES_HERE
  dout : Outport  OutDataType=sfix(16)  OutScaling=2^0
  wires:
  Constant1/1 -> Addressable Shift Register/2
  Addressable Shift Register/1 -> dout/1
  din/1 -> Addressable Shift Register/1

== system xrbsComm_r4/White Gaussian  Noise Generator/Box-Muller2/fr1/lfsr_29_2/x8/ASR ==
  din : Inport  OutDataType=sfix(16)  OutScaling=2^0
  Addressable Shift Register : xbsIndex_r4/Addressable Shift Register  infer_latency=off  depth=asr_length  initVector=init  en=off  dbl_ovrd=off  use_behavioral_HDL=off  use_rpm=off  block_type=addrsr
      settings: infoedit="Delay of configurable length.  Any element in the delay line can be addressed and driven onto the output port.<P><P>Hardware notes: Implemented using SRL16s.  If a Virtex-II device is used, multiple SRLC16s are cascaded together."  xl_area=[0, 0, 0, 0, 0, 0, 0]  block_version=VER_STRING_GOES_HERE
  Constant1 : xbsIndex_r4/Constant  arith_type=Unsigned  const=asr_length-1  n_bits=size(dec2bin(asr_length-1),2)  bin_pt=0  explicit_period=off  period=1  equ=P=C  opselect=C  inp2=PCIN>>17  opr=+  inp1=P  carry=CIN  dbl_ovrd=off  block_type=constant
      settings: block_version=VER_STRING_GOES_HERE
  dout : Outport  OutDataType=sfix(16)  OutScaling=2^0
  wires:
  Constant1/1 -> Addressable Shift Register/2
  Addressable Shift Register/1 -> dout/1
  din/1 -> Addressable Shift Register/1

== system xrbsComm_r4/White Gaussian  Noise Generator/Box-Muller2/fr1/lfsr_31_2/x5/ASR ==
  din : Inport  OutDataType=sfix(16)  OutScaling=2^0
  Addressable Shift Register : xbsIndex_r4/Addressable Shift Register  infer_latency=off  depth=asr_length  initVector=init  en=off  dbl_ovrd=off  use_behavioral_HDL=off  use_rpm=off  block_type=addrsr
      settings: infoedit="Delay of configurable length.  Any element in the delay line can be addressed and driven onto the output port.<P><P>Hardware notes: Implemented using SRL16s.  If a Virtex-II device is used, multiple SRLC16s are cascaded together."  xl_area=[0, 0, 0, 0, 0, 0, 0]  block_version=VER_STRING_GOES_HERE
  Constant1 : xbsIndex_r4/Constant  arith_type=Unsigned  const=asr_length-1  n_bits=size(dec2bin(asr_length-1),2)  bin_pt=0  explicit_period=off  period=1  equ=P=C  opselect=C  inp2=PCIN>>17  opr=+  inp1=P  carry=CIN  dbl_ovrd=off  block_type=constant
      settings: block_version=VER_STRING_GOES_HERE
  dout : Outport  OutDataType=sfix(16)  OutScaling=2^0
  wires:
  Constant1/1 -> Addressable Shift Register/2
  Addressable Shift Register/1 -> dout/1
  din/1 -> Addressable Shift Register/1

== system xrbsComm_r4/White Gaussian  Noise Generator/Box-Muller2/fr1/lfsr_31_2/x6/ASR ==
  din : Inport  OutDataType=sfix(16)  OutScaling=2^0
  Addressable Shift Register : xbsIndex_r4/Addressable Shift Register  infer_latency=off  depth=asr_length  initVector=init  en=off  dbl_ovrd=off  use_behavioral_HDL=off  use_rpm=off  block_type=addrsr
      settings: infoedit="Delay of configurable length.  Any element in the delay line can be addressed and driven onto the output port.<P><P>Hardware notes: Implemented using SRL16s.  If a Virtex-II device is used, multiple SRLC16s are cascaded together."  xl_area=[0, 0, 0, 0, 0, 0, 0]  block_version=VER_STRING_GOES_HERE
  Constant1 : xbsIndex_r4/Constant  arith_type=Unsigned  const=asr_length-1  n_bits=size(dec2bin(asr_length-1),2)  bin_pt=0  explicit_period=off  period=1  equ=P=C  opselect=C  inp2=PCIN>>17  opr=+  inp1=P  carry=CIN  dbl_ovrd=off  block_type=constant
      settings: block_version=VER_STRING_GOES_HERE
  dout : Outport  OutDataType=sfix(16)  OutScaling=2^0
  wires:
  Constant1/1 -> Addressable Shift Register/2
  Addressable Shift Register/1 -> dout/1
  din/1 -> Addressable Shift Register/1
